simulink model "regulator_dyskretny"  (R2013b)
settings: Solver=ode3  StartTime=0.0  StopTime=500  FixedStep=0.1  RelTol=1e-3
values from neighbouring files (symbols this model uses):
  a = 31    [charakterystyka_pompa.m]    (also in charakterystyka_pompa_sterownik.m; dane14listopad.mat; danePompa.mat; pomiary.m)
  b = 40    [charakterystyki_zawory_reczne.m]    (also in daneZawory_cz2.mat; pomiary.m; rhs.m)
  c = p(1)    [cel.m]    (also in charakterystyki_zawory_reczne.m = 10; daneZawory_cz2.mat = 10; identyfikacja_parametrow.m = 10; identyfikacja_zawor2.m = 10)
  C1 = q/sqrt(H1pp)    [linearyzacja_analitycznie.m]    (also in wskaznikZawor1.m = parametry(1))
  C2 = q/sqrt(H2pp)    [linearyzacja_analitycznie.m]    (also in wskaznikZawor2.m = parametry(1))
  C3 = q/sqrt(H3pp)    [linearyzacja_analitycznie.m]    (also in wskaznikZawor3.m = parametry(1))
  H2max = 40    [charakterystyki_zawory_reczne.m]    (also in daneZawory_cz2.mat; pomiary.m)
  K = [0.0311 0.0151 0.0068]    [testy_regulatora.m]    (also in wagiLQ.m = K_par)
  R = 40    [charakterystyki_zawory_reczne.m]    (also in daneZawory_cz2.mat; nastawyLQ.m; pomiary.m; rhs.m)
  w = 5    [charakterystyka_pompa.m]    (also in charakterystyka_pompa_sterownik.m; dane14listopad.mat; danePompa.mat; pomiary.m)
  x = max(x,0)    [rhs.m]
settings Model: Creator=Michal  LastModifiedBy=Michal

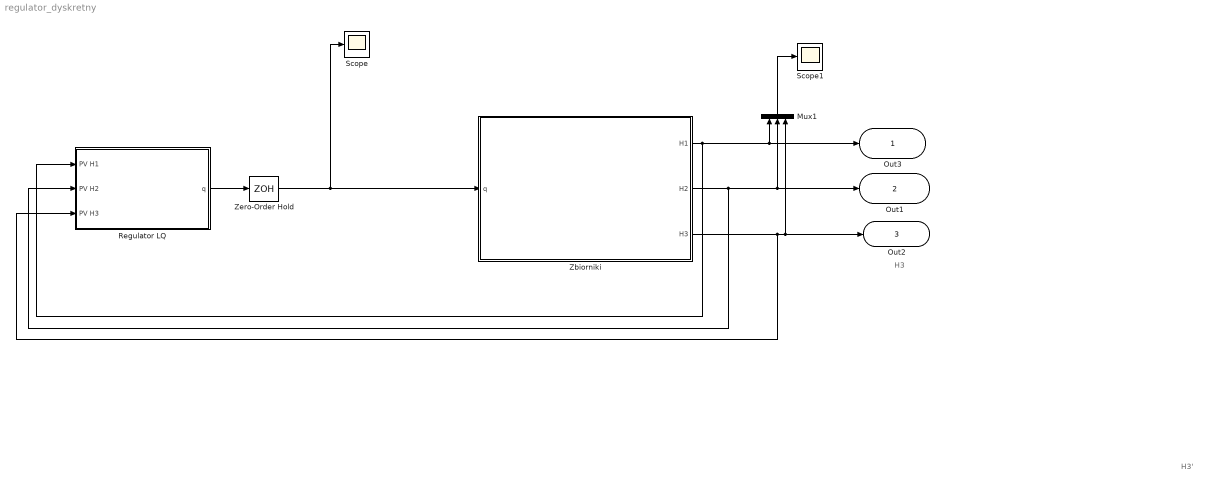
== system regulator_dyskretny ==
  note: H3
  note: H3'
  Mux1 : Mux  Inputs=3
  Regulator LQ : Subsystem
  Scope : Scope
      settings: TimeRange=500  SaveName=q_lqr
  Scope1 : Scope
      settings: TimeRange=500  YMin=-300000  YMax=50000  SaveName=H_lqr
  Zbiorniki : Subsystem
  Zero-Order Hold : ZeroOrderHold  SampleTime=0.1
  Out3 : Outport
  Out1 : Outport  Port=2
  Out2 : Outport  Port=3
  wires:
  Zbiorniki/3(H3) -> Regulator LQ/3(PV H3), Out2/1, Mux1/3
  Zbiorniki/1(H1) -> Regulator LQ/1(PV H1), Mux1/1, Out3/1
  Zbiorniki/2(H2) -> Regulator LQ/2(PV H2), Mux1/2, Out1/1
  Mux1/1 -> Scope1/1
  Regulator LQ/1(q) -> Zero-Order Hold/1
  Zero-Order Hold/1 -> Scope/1, Zbiorniki/1(q)

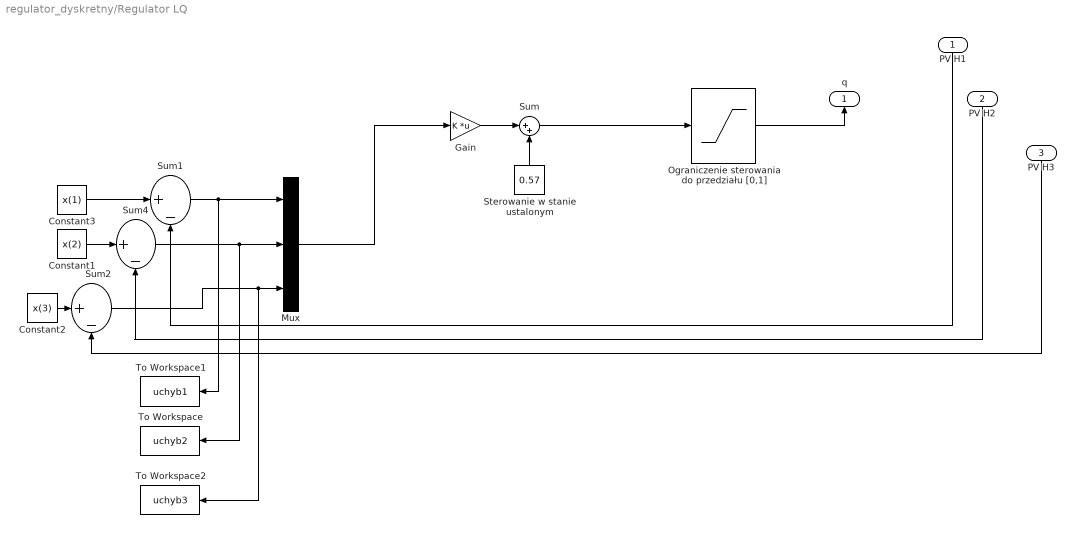
== system regulator_dyskretny/Regulator LQ ==
  PV H1 : Inport
  PV H2 : Inport  Port=2
  PV H3 : Inport  Port=3
  Constant1 : Constant  Value=x(2)
  Constant2 : Constant  Value=x(3)
  Constant3 : Constant  Value=x(1)
  Gain : Gain  Gain=K  Multiplication=Matrix(K*u)
  Mux : Mux  Inputs=3
  Ograniczenie sterowania do przedziału [0,1] : Saturate  UpperLimit=1  LowerLimit=0
  Sterowanie w stanie ustalonym : Constant  Value=0.57
  Sum : Sum  Inputs=|++
  Sum1 : Sum  Inputs=|+-
  Sum2 : Sum  Inputs=|+-
  Sum4 : Sum  Inputs=|+-
  To Workspace : ToWorkspace  VariableName=uchyb2  SampleTime=-1  SaveFormat=Structure With Time
  To Workspace1 : ToWorkspace  VariableName=uchyb1  SampleTime=-1  SaveFormat=Structure With Time
  To Workspace2 : ToWorkspace  VariableName=uchyb3  SampleTime=-1  SaveFormat=Structure With Time
  q : Outport
  wires:
  PV H1/1 -> Sum1/2
  PV H3/1 -> Sum2/2
  PV H2/1 -> Sum4/2
  Sum1/1 -> To Workspace1/1, Mux/1
  Sum2/1 -> To Workspace2/1, Mux/3
  Sum4/1 -> To Workspace/1, Mux/2
  Constant2/1 -> Sum2/1
  Constant1/1 -> Sum4/1
  Constant3/1 -> Sum1/1
  Sterowanie w stanie ustalonym/1 -> Sum/2
  Ograniczenie sterowania do przedziału [0,1]/1 -> q/1
  Sum/1 -> Ograniczenie sterowania do przedziału [0,1]/1
  Gain/1 -> Sum/1
  Mux/1 -> Gain/1

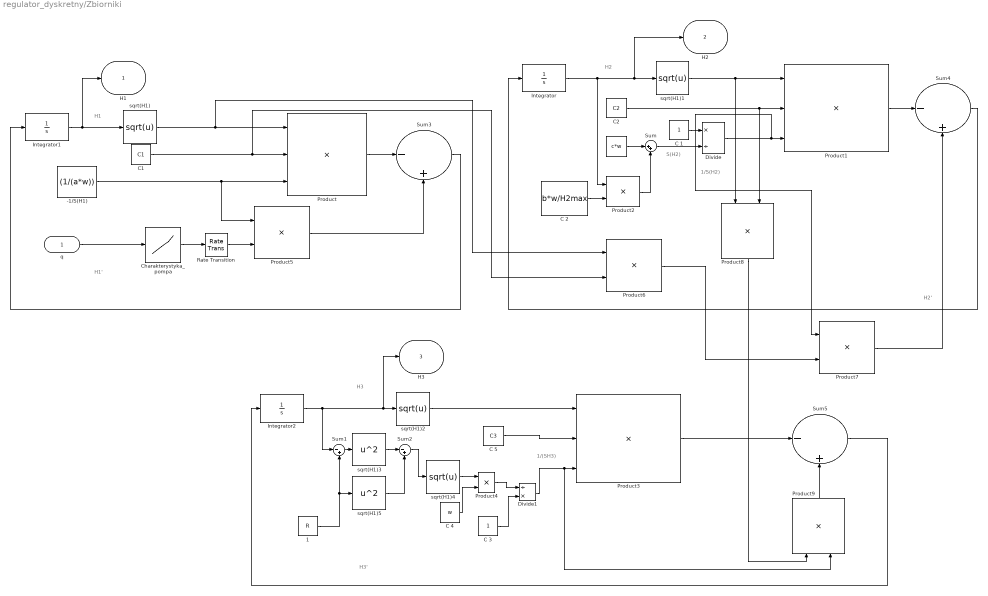
== system regulator_dyskretny/Zbiorniki ==
  note: H1
  note: 1/S(H2)
  note: S(H2)
  note: H2'
  note: H2
  note: 1/(SH3)
  note: H3
  note: H1'
  note: H3'
  q : Inport
  " " : Constant  Value=c*w
  " 1" : Constant  Value=R
  -1/S(H1) : Constant  Value=(1/(a*w))
  C 1 : Constant
  C 2 : Constant  Value=b*w/H2max
  C 3 : Constant
  C 4 : Constant  Value=w
  C 5 : Constant  Value=C3
  "C1 " : Constant  Value=C1
  "C2 " : Constant  Value=C2
  Charakterystyka_pompa : Lookup_n-D  NumberOfTableDimensions=1  BreakpointsForDimension1="[0.180000000000000\t0.181000000000000\t0.182000000000000\t0.183000000000000\t0.184000000000000\t0.185000000000000\t0.186000000000000\t0.187000000000000\t0.188000000000000\t0.189000000000000\t0.190000000000000\t0.191000000000000\t0.192000000000000\t0.193000000000000\t0.194000000000000\t0.195000000000000\t0.196000000000000\t0.197000000000000\t0.198000000000000\t0.199000000000000\t0.200000000000000\t0.201000000000000\t0.202000000000000\t0.203000000000000\t0.204000000000000\t0.205000000000000\t0.206000000000000\t0.207000000000000\t0.208000000000000\t0.209000000000000\t0.210000000000000\t0.211000000000000\t0.212000000000000\t0.213000000000000\t0.214000000000000\t0.215000000000000\t0.216000000000000\t0.217000000000000\t0.218000000000000\t0.219000000000000\t0.220000000000000\t0.221000000000000\t0.222000000000000\t0.223000000000000\t0.224000000000000\t0.225000000000000\t0.226000000000000\t0.227000000000000\t0.228000000000000\t0.229000000000000\t0.230000000000000\t0.231000000000000\t0.232000000000000\t0.233000000000000\t0.234000000000000\t0.235000000000000\t0.236000000000000\t0.237000000000000\t0.238000000000000\t0.239000000000000\t0.240000000000000\t0.241000000000000\t0.242000000000000\t0.243000000000000\t0.244000000000000\t0.245000000000000\t0.246000000000000\t0.247000000000000\t0.248000000000000\t0.249000000000000\t0.250000000000000\t0.251000000000000\t0.252000000000000\t0.253000000000000\t0.254000000000000\t0.255000000000000\t0.256000000000000\t0.257000000000000\t0.258000000000000\t0.259000000000000\t0.260000000000000\t0.261000000000000\t0.262000000000000\t0.263000000000000\t0.264000000000000\t0.265000000000000\t0.266000000000000\t0.267000000000000\t0.268000000000000\t0.269000000000000\t0.270000000000000\t0.271000000000000\t0.272000000000000\t0.273000000000000\t0.274000000000000\t0.275000000000000\t0.276000000000000\t0.277000000000000\t0.278000000000000\t0.279000000000000\t0.280000000000000\t0.281000000000000\t0.282000000000000\t0.283000000000000\t0.284000000000000\t0.285000000000000\t0.286000000000000\t0.287000000000000\t0.288000000000000\t0.289000000000000\t0.290000000000000\t0.291000000000000\t0.292000000000000\t0.293000000000000\t0.294000000000000\t0.295000000000000\t0.296000000000000\t0.297000000000000\t0.298000000000000\t0.299000000000000\t0.300000000000000\t0.301000000000000\t0.302000000000000\t0.303000000000000\t0.304000000000000\t0.305000000000000\t0.306000000000000\t0.307000000000000\t0.308000000000000\t0.309000000000000\t0.310000000000000\t0.311000000000000\t0.312000000000000\t0.313000000000000\t0.314000000000000\t0.315000000000000\t0.316000000000000\t0.317000000000000\t0.318000000000000\t0.319000000000000\t0.320000000000000\t0.321000000000000\t0.322000000000000\t0.323000000000000\t0.324000000000000\t0.325000000000000\t0.326000000000000\t0.327000000000000\t0.328000000000000\t0.329000000000000\t0.330000000000000\t0.331000000000000\t0.332000000000000\t0.333000000000000\t0.334000000000000\t0.335000000000000\t0.336000000000000\t0.337000000000000\t0.338000000000000\t0.339000000000000\t0.340000000000000\t0.341000000000000\t0.342000000000000\t0.343000000000000\t0.344000000000000\t0.345000000000000\t0.346000000000000\t0.347000000000000\t0.348000000000000\t0.349000000000000\t0.350000000000000\t0.351000000000000\t0.352000000000000\t0.353000000000000\t0.354000000000000\t0.355000000000000\t0.356000000000000\t0.357000000000000\t0.358000000000000\t0.359000000000000\t0.360000000000000\t0.361000000000000\t0.362000000000000\t0.363000000000000\t0.364000000000000\t0.365000000000000\t0.366000000000000\t0.367000000000000\t0.368000000000000\t0.369000000000000\t0.370000000000000\t0.371000000000000\t0.372000000000000\t0.373000000000000\t0.374000000000000\t0.375000000000000\t0.376000000000000\t0.377000000000000\t0.378000000000000\t0.379000000000000\t0.380000000000000\t0.381000000000000\t0.382000000000000\t0.383000000000000\t0.384000000000000\t0.385000000000000\t0.386000000000000\t0.387000000000000\t0.388000000000000\t0.389000000000000\t0.390000000000000\t0.391000000000000\t0.392000000000000\t0.393000000000000\t0.394000000000000\t0.395000000000000\t0.396000000000000\t0.397000000000000\t0.398000000000000\t0.399000000000000\t0.400000000000000\t0.401000000000000\t0.402000000000000\t0.403000000000000\t0.404000000000000\t0.405000000000000\t0.406000000000000\t0.407000000000000\t0.408000000000000\t0.409000000000000\t0.410000000000000\t0.411000000000000\t0.412000000000000\t0.413000000000000\t0.414000000000000\t0.415000000000000\t0.416000000000000\t0.417000000000000\t0.418000000000000\t0.419000000000000\t0.420000000000000\t0.421000000000000\t0.422000000000000\t0.423000000000000\t0.424000000000000\t0.425000000000000\t0.426000000000000\t0.427000000000000\t0.428000000000000\t0.429000000000000\t0.430000000000000\t0.431000000000000\t0.432000000000000\t0.433000000000000\t0.434000000000000\t0.435000000000000\t0.436000000000000\t0.437000000000000\t0.438000000000000\t0.439000000000000\t0.440000000000000\t0.441000000000000\t0.442000000000000\t0.443000000000000\t0.444000000000000\t0.445000000000000\t0.446000000000000\t0.447000000000000\t0.448000000000000\t0.449000000000000\t0.450000000000000\t0.451000000000000\t0.452000000000000\t0.453000000000000\t0.454000000000000\t0.455000000000000\t0.456000000000000\t0.457000000000000\t0.458000000000000\t0.459000000000000\t0.460000000000000\t0.461000000000000\t0.462000000000000\t0.463000000000000\t0.464000000000000\t0.465000000000000\t0.466000000000000\t0.467000000000000\t0.468000000000000\t0.469000000000000\t0.470000000000000\t0.471000000000000\t0.472000000000000\t0.473000000000000\t0.474000000000000\t0.475000000000000\t0.476000000000000\t0.477000000000000\t0.478000000000000\t0.479000000000000\t0.480000000000000\t0.481000000000000\t0.482000000000000\t0.483000000000000\t0.484000000000000\t0.485000000000000\t0.486000000000000\t0.487000000000000\t0.488000000000000\t0.489000000000000\t0.490000000000000\t0.491000000000000\t0.492000000000000\t0.493000000000000\t0.494000000000000\t0.495000000000000\t0.496000000000000\t0.497000000000000\t0.498000000000000\t0.499000000000000\t0.500000000000000\t0.501000000000000\t0.502000000000000\t0.503000000000000\t0.504000000000000\t0.505000000000000\t0.506000000000000\t0.507000000000000\t0.508000000000000\t0.509000000000000\t0.510000000000000\t0.511000000000000\t0.512000000000000\t0.513000000000000\t0.514000000000000\t0.515000000000000\t0.516000000000000\t0.517000000000000\t0.518000000000000\t0.519000000000000\t0.520000000000000\t0.521000000000000\t0.522000000000000\t0.523000000000000\t0.524000000000000\t0.525000000000000\t0.526000000000000\t0.527000000000000\t0.528000000000000\t0.529000000000000\t0.530000000000000\t0.531000000000000\t0.532000000000000\t0.533000000000000\t0.534000000000000\t0.535000000000000\t0.536000000000000\t0.537000000000000\t0.538000000000000\t0.539000000000000\t0.540000000000000\t0.541000000000000\t0.542000000000000\t0.543000000000000\t0.544000000000000\t0.545000000000000\t0.546000000000000\t0.547000000000000\t0.548000000000000\t0.549000000000000\t0.550000000000000\t0.551000000000000\t0.552000000000000\t0.553000000000000\t0.554000000000000\t0.555000000000000\t0.556000000000000\t0.557000000000000\t0.558000000000000\t0.559000000000000\t0.560000000000000\t0.561000000000000\t0.562000000000000\t0.563000000000000\t0.564000000000000\t0.565000000000000\t0.566000000000000\t0.567000000000000\t0.568000000000000\t0.569000000000000\t0.570000000000000\t0.571000000000000\t0.572000000000000\t0.573000000000000\t0.574000000000000\t0.575000000000000\t0.576000000000000\t0.577000000000000\t0.578000000000000\t0.579000000000000\t0.580000000000000\t0.581000000000000\t0.582000000000000\t0.583000000000000\t0.584000000000000\t0.585000000000000\t0.586000000000000\t0.587000000000000\t0.588000000000000\t0.589000000000000\t0.590000000000000\t0.591000000000000\t0.592000000000000\t0.593000000000000\t0.594000000000000\t0.595000000000000\t0.596000000000000\t0.597000000000000\t0.598000000000000\t0.599000000000000\t0.600000000000000\t0.601000000000000\t0.602000000000000\t0.603000000000000\t0.604000000000000\t0.605000000000000\t0.606000000000000\t0.607000000000000\t0.608000000000000\t0.609000000000000\t0.610000000000000\t0.611000000000000\t0.612000000000000\t0.613000000000000\t0.614000000000000\t0.615000000000000\t0.616000000000000\t0.617000000000000\t0.618000000000000\t0.619000000000000\t0.620000000000000\t0.621000000000000\t0.622000000000000\t0.623000000000000\t0.624000000000000\t0.625000000000000\t0.626000000000000\t0.627000000000000\t0.628000000000000\t0.629000000000000\t0.630000000000000\t0.631000000000000\t0.632000000000000\t0.633000000000000\t0.634000000000000\t0.635000000000000\t0.636000000000000\t0.637000000000000\t0.638000000000000\t0.639000000000000\t0.640000000000000\t0.641000000000000\t0.642000000000000\t0.643000000000000\t0.644000000000000\t0.645000000000000\t0.646000000000000\t0.647000000000000\t0.648000000000000\t0.649000000000000\t0.650000000000000\t0.651000000000000\t0.652000000000000\t0.653000000000000\t0.654000000000000\t0.655000000000000\t0.656000000000000\t0.657000000000000\t0.658000000000000\t0.659000000000000\t0.660000000000000\t0.661000000000000\t0.662000000000000\t0.663000000000000\t0.664000000000000\t0.665000000000000\t0.666000000000000\t0.667000000000000\t0.668000000000000\t0.669000000000000\t0.670000000000000\t0.671000000000000\t0.672000000000000\t0.673000000000000\t0.674000000000000\t0.675000000000000\t0.676000000000000\t0.677000000000000\t0.678000000000000\t0.679000000000000\t0.680000000000000\t0.681000000000000\t0.682000000000000\t0.683000000000000\t0.684000000000000\t0.685000000000000\t0.686000000000000\t0.687000000000000\t0.688000000000000\t0.689000000000000\t0.690000000000000\t0.691000000000000\t0.692000000000000\t0.693000000000000\t0.694000000000000\t0.695000000000000\t0.696000000000000\t0.697000000000000\t0.698000000000000\t0.699000000000000\t0.700000000000000\t0.701000000000000\t0.702000000000000\t0.703000000000000\t0.704000000000000\t0.705000000000000\t0.706000000000000\t0.707000000000000\t0.708000000000000\t0.709000000000000\t0.710000000000000\t0.711000000000000\t0.712000000000000\t0.713000000000000\t0.714000000000000\t0.715000000000000\t0.716000000000000\t0.717000000000000\t0.718000000000000\t0.719000000000000\t0.720000000000000\t0.721000000000000\t0.722000000000000\t0.723000000000000\t0.724000000000000\t0.725000000000000\t0.726000000000000\t0.727000000000000\t0.728000000000000\t0.729000000000000\t0.730000000000000\t0.731000000000000\t0.732000000000000\t0.733000000000000\t0.734000000000000\t0.735000000000000\t0.736000000000000\t0.737000000000000\t0.738000000000000\t0.739000000000000\t0.740000000000000\t0.741000000000000\t0.742000000000000\t0.743000000000000\t0.744000000000000\t0.745000000000000\t0.746000000000000\t0.747000000000000\t0.748000000000000\t0.749000000000000\t0.750000000000000\t0.751000000000000\t0.752000000000000\t0.753000000000000\t0.754000000000000\t0.755000000000000\t0.756000000000000\t0.757000000000000\t0.758000000000000\t0.759000000000000\t0.760000000000000\t0.761000000000000\t0.762000000000000\t0.763000000000000\t0.764000000000000\t0.765000000000000\t0.766000000000000\t0.767000000000000\t0.768000000000000\t0.769000000000000\t0.770000000000000\t0.771000000000000\t0.772000000000000\t0.773000000000000\t0.774000000000000\t0.775000000000000\t0.776000000000000\t0.777000000000000\t0.778000000000000\t0.779000000000000\t0.780000000000000\t0.781000000000000\t0.782000000000000\t0.783000000000000\t0.784000000000000\t0.785000000000000\t0.786000000000000\t0.787000000000000\t0.788000000000000\t0.789000000000000\t0.790000000000000\t0.791000000000000\t0.792000000000000\t0.793000000000000\t0.794000000000000\t0.795000000000000\t0.796000000000000\t0.797000000000000\t0.798000000000000\t0.799000000000000\t0.800000000000000\t0.801000000000000\t0.802000000000000\t0.803000000000000\t0.804000000000000\t0.805000000000000\t0.806000000000000\t0.807000000000000\t0.808000000000000\t0.809000000000000\t0.810000000000000\t0.811000000000000\t0.812000000000000\t0.813000000000000\t0.814000000000000\t0.815000000000000\t0.816000000000000\t0.817000000000000\t0.818000000000000\t0.819000000000000\t0.820000000000000\t0.821000000000000\t0.822000000000000\t0.823000000000000\t0.824000000000000\t0.825000000000000\t0.826000000000000\t0.827000000000000\t0.828000000000000\t0.829000000000000\t0.830000000000000\t0.831000000000000\t0.832000000000000\t0.833000000000000\t0.834000000000000\t0.835000000000000\t0.836000000000000\t0.837000000000000\t0.838000000000000\t0.839000000000000\t0.840000000000000\t0.841000000000000\t0.842000000000000\t0.843000000000000\t0.844000000000000\t0.845000000000000\t0.846000000000000\t0.847000000000000\t0.848000000000000\t0.849000000000000\t0.850000000000000\t0.851000000000000\t0.852000000000000\t0.853000000000000\t0.854000000000000\t0.855000000000000\t0.856000000000000\t0.857000000000000\t0.858000000000000\t0.859000000000000\t0.860000000000000\t0.861000000000000\t0.862000000000000\t0.863000000000000\t0.864000000000000\t0.865000000000000\t0.866000000000000\t0.867000000000000\t0.868000000000000\t0.869000000000000\t0.870000000000000\t0.871000000000000\t0.872000000000000\t0.873000000000000\t0.874000000000000\t0.875000000000000\t0.876000000000000\t0.877000000000000\t0.878000000000000\t0.879000000000000\t0.880000000000000\t0.881000000000000\t0.882000000000000\t0.883000000000000\t0.884000000000000\t0.885000000000000\t0.886000000000000\t0.887000000000000\t0.888000000000000\t0.889000000000000\t0.890000000000000\t0.891000000000000\t0.892000000000000\t0.893000000000000\t0.894000000000000\t0.895000000000000\t0.896000000000000\t0.897000000000000\t0.898000000000000\t0.899000000000000\t0.900000000000000\t0.901000000000000\t0.902000000000000\t0.903000000000000\t0.904000000000000\t0.905000000000000\t0.906000000000000\t0.907000000000000\t0.908000000000000\t0.909000000000000\t0.910000000000000\t0.911000000000000\t0.912000000000000\t0.913000000000000\t0.914000000000000\t0.915000000000000\t0.916000000000000\t0.917000000000000\t0.918000000000000\t0.919000000000000\t0.920000000000000\t0.921000000000000\t0.922000000000000\t0.923000000000000\t0.924000000000000\t0.925000000000000\t0.926000000000000\t0.927000000000000\t0.928000000000000\t0.929000000000000\t0.930000000000000\t0.931000000000000\t0.932000000000000\t0.933000000000000\t0.934000000000000\t0.935000000000000\t0.936000000000000\t0.937000000000000\t0.938000000000000\t0.939000000000000\t0.940000000000000\t0.941000000000000\t0.942000000000000\t0.943000000000000\t0.944000000000000\t0.945000000000000\t0.946000000000000\t0.947000000000000\t0.948000000000000\t0.949000000000000\t0.950000000000000\t0.951000000000000\t0.952000000000000\t0.953000000000000\t0.954000000000000\t0.955000000000000\t0.956000000000000\t0.957000000000000\t0.958000000000000\t0.959000000000000\t0.960000000000000\t0.961000000000000\t0.962000000000000\t0.963000000000000\t0.964000000000000\t0.965000000000000\t0.966000000000000\t0.967000000000000\t0.968000000000000\t0.969000000000000\t0.970000000000000\t0.971000000000000\t0.972000000000000\t0.973000000000000\t0.974000000000000\t0.975000000000000\t0.976000000000000\t0.977000000000000\t0.978000000000000\t0.979000000000000\t0.980000000000000\t0.981000000000000\t0.982000000000000\t0.983000000000000\t0.984000000000000\t0.985000000000000\t0.986000000000000\t0.987000000000000\t0.988000000000000\t0.989000000000000\t0.990000000000000\t0.991000000000000\t0.992000000000000\t0.993000000000000\t0.994000000000000\t0.995000000000000\t0.996000000000000\t0.997000000000000\t0.998000000000000\t0.999000000000000\t1]"  Table="[12.0028336476540\t12.3293606666216\t12.6550486652732\t12.9798992380227\t13.3039139792839\t13.6270944834709\t13.9494423449973\t14.2709591582772\t14.5916465177244\t14.9115060177528\t15.2305392527763\t15.5487478172088\t15.8661333054640\t16.1826973119561\t16.4984414310987\t16.8133672573059\t17.1274763849915\t17.4407704085693\t17.7532509224533\t18.0649195210574\t18.3757777987953\t18.6858273500811\t18.9950697693286\t19.3035066509517\t19.6111395893642\t19.9179701789801\t20.2240000142132\t20.5292306894775\t20.8336637991868\t21.1373009377549\t21.4401436995959\t21.7421936791235\t22.0434524707516\t22.3439216688942\t22.6436028679651\t22.9424976623782\t23.2406076465474\t23.5379344148866\t23.8344795618096\t24.1302446817304\t24.4252313690628\t24.7194412182207\t25.0128758236180\t25.3055367796686\t25.5974256807863\t25.8885441213852\t26.1788936958789\t26.4684759986814\t26.7572926242067\t27.0453451668686\t27.3326352210809\t27.6191643812576\t27.9049342418125\t28.1899463971596\t28.4742024417127\t28.7577039698856\t29.0404525760924\t29.3224498547468\t29.6036974002628\t29.8841968070542\t30.1639496695350\t30.4429575821190\t30.7212221392200\t30.9987449352520\t31.2755275646289\t31.5515716217645\t31.8268787010728\t32.1014503969676\t32.3752883038628\t32.6483940161723\t32.9207691283099\t33.1924152346896\t33.4633339297253\t33.7335268078307\t34.0029954634199\t34.2717414909067\t34.5397664847049\t34.8070720392286\t35.0736597488914\t35.3395312081074\t35.6046880112905\t35.8691317528544\t36.1328640272131\t36.3958864287805\t36.6582005519705\t36.9198079911969\t37.1807103408736\t37.4409091954146\t37.7004061492336\t37.9592027967446\t38.2173007323615\t38.4747015504981\t38.7314068455684\t38.9874182119862\t39.2427372441654\t39.4973655365200\t39.7513046834636\t40.0045562794104\t40.2571219187741\t40.5090031959686\t40.7602017054078\t41.0107190415057\t41.2605567986760\t41.5097165713327\t41.7581999538896\t42.0060085407607\t42.2531439263599\t42.4996077051009\t42.7454014713977\t42.9905268196642\t43.2349853443143\t43.4787786397618\t43.7219083004207\t43.9643759207047\t44.2061830950279\t44.4473314178040\t44.6878224834471\t44.9276578863709\t45.1668392209893\t45.4053680817163\t45.6432460629656\t45.8804747591513\t46.1170557646872\t46.3529906739871\t46.5882810814650\t46.8229285815347\t47.0569347686101\t47.2903012371052\t47.5230295814337\t47.7551213960096\t47.9865782752468\t48.2174018135591\t48.4475936053605\t48.6771552450647\t48.9060883270858\t49.1343944458375\t49.3620751957338\t49.5891321711886\t49.8155669666157\t50.0413811764291\t50.2665763950425\t50.4911542168699\t50.7151162363253\t50.9384640478223\t51.1611992457751\t51.3833234245973\t51.6048381787030\t51.8257451025060\t52.0460457904202\t52.2657418368594\t52.4848348362376\t52.7033263829687\t52.9212180714665\t53.1385114961448\t53.3552082514177\t53.5713099316990\t53.7868181314025\t54.0017344449422\t54.2160604667319\t54.4297977911855\t54.6429480127170\t54.8555127257401\t55.0674935246688\t55.2788920039170\t55.4897097578985\t55.6999483810273\t55.9096094677171\t56.1186946123820\t56.3272054094357\t56.5351434532922\t56.7425103383654\t56.9493076590691\t57.1555370098172\t57.3611999850236\t57.5662981791023\t57.7708331864670\t57.9748066015317\t58.1782200187102\t58.3810750324164\t58.5833732370643\t58.7851162270677\t58.9863055968404\t59.1869429407965\t59.3870298533496\t59.5865679289139\t59.7855587619030\t59.9840039467310\t60.1819050778117\t60.3792637495589\t60.5760815563866\t60.7723600927087\t60.9681009529389\t61.1633057314914\t61.3579760227798\t61.5521134212181\t61.7457195212202\t61.9387959171999\t62.1313442035712\t62.3233659747479\t62.5148628251439\t62.7058363491732\t62.8962881412495\t63.0862197957868\t63.2756329071989\t63.4645290698998\t63.6529098783032\t63.8407769268232\t64.0281318098736\t64.2149761218683\t64.4013114572211\t64.5871394103460\t64.7724615756568\t64.9572795475674\t65.1415949204918\t65.3254092888437\t65.5087242470371\t65.6915413894858\t65.8738623106038\t66.0556886048049\t66.2370218665030\t66.4178636901120\t66.5982156700458\t66.7780794007183\t66.9574564765433\t67.1363484919347\t67.3147570413065\t67.4926837190724\t67.6701301196465\t67.8470978374425\t68.0235884668744\t68.1996036023560\t68.3751448383013\t68.5502137691241\t68.7248119892382\t68.8989410930576\t69.0726026749963\t69.2457983294680\t69.4185296508865\t69.5907982336660\t69.7626056722201\t69.9339535609629\t70.1048434943080\t70.2752770666696\t70.4452558724614\t70.6147815060973\t70.7838555619913\t70.9524796345572\t71.1206553182088\t71.2883842073601\t71.4556678964250\t71.6225079798173\t71.7889060519509\t71.9548637072397\t72.1203825400977\t72.2854641449386\t72.4501101161764\t72.6143220482249\t72.7781015354980\t72.9414501724097\t73.1043695533738\t73.2668612728042\t73.4289269251147\t73.5905681047193\t73.7517864060318\t73.9125834234662\t74.0729607514363\t74.2329199843560\t74.3924627166392\t74.5515905426997\t74.7103050569515\t74.8686078538084\t75.0265005276843\t75.1839846729932\t75.3410618841488\t75.4977337555651\t75.6540018816559\t75.8098678568353\t75.9653332755169\t76.1203997321148\t76.2750688210427\t76.4293421367147\t76.5832212735445\t76.7367078259461\t76.8898033883332\t77.0425095551200\t77.1948279207201\t77.3467600795475\t77.4983076260161\t77.6494721545398\t77.8002552595325\t77.9506585354079\t78.1006835765800\t78.2503319774628\t78.3996053324701\t78.5485052360157\t78.6970332825136\t78.8451910663776\t78.9929801820217\t79.1404022238596\t79.2874587863054\t79.4341514637729\t79.5804818506758\t79.7264515414283\t79.8720621304441\t80.0173152121371\t80.1622123809213\t80.3067552312104\t80.4509453574184\t80.5947843539591\t80.7382738152465\t80.8814153356944\t81.0242105097167\t81.1666609317274\t81.3087681961402\t81.4505338973690\t81.5919596298279\t81.7330469879306\t81.8737975660909\t82.0142129587229\t82.1542947602405\t82.2940445650573\t82.4334639675875\t82.5725545622448\t82.7113179434431\t82.8497557055963\t82.9878694431183\t83.1256607504231\t83.2631312219243\t83.4002824520361\t83.5371160351722\t83.6736335657465\t83.8098366381729\t83.9457268468653\t84.0813057862376\t84.2165750507037\t84.3515362346774\t84.4861909325726\t84.6205407388033\t84.7545872477833\t84.8883320539264\t85.0217767516467\t85.1549229353579\t85.2877721994739\t85.4203261384087\t85.5525863465760\t85.6845544183899\t85.8162319482642\t85.9476205306127\t86.0787217598494\t86.2095372303881\t86.3400685366427\t86.4703172730272\t86.6002850339553\t86.7299734138410\t86.8593840070982\t86.9885184081407\t87.1173782113825\t87.2459650112374\t87.3742804021192\t87.5023259784420\t87.6301033346195\t87.7576140650657\t87.8848597641944\t88.0118420264195\t88.1385624461550\t88.2650226178146\t88.3912241358123\t88.5171685945621\t88.6428575884776\t88.7682927119728\t88.8934755594617\t89.0184077253581\t89.1430908040759\t89.2675263900290\t89.3917160776312\t89.5156614612964\t89.6393641354386\t89.7628256944716\t89.8860477328093\t90.0090318448656\t90.1317796250543\t90.2542926677894\t90.3765725674847\t90.4986209185542\t90.6204393154117\t90.7420293524710\t90.8633926241461\t90.9845307248509\t91.1054452489992\t91.2261377910050\t91.3466099452821\t91.4668633062444\t91.5868994683057\t91.7067200258800\t91.8263265733812\t91.9457207052231\t92.0649040158197\t92.1838780995847\t92.3026445509322\t92.4212049642759\t92.5395609340298\t92.6577140546077\t92.7756659204236\t92.8934181258913\t93.0109722654247\t93.1283299334376\t93.2454927243441\t93.3624622325579\t93.4792400524930\t93.5958277785631\t93.7122270051823\t93.8284393267644\t93.9444663377232\t94.0603096324728\t94.1759708054268\t94.2914514509994\t94.4067531636042\t94.5218775376552\t94.6368261675664\t94.7516006477515\t94.8662025726245\t94.9806335365991\t95.0948951340895\t95.2089889595093\t95.3229166072726\t95.4366796717931\t95.5502797474848\t95.6637184287616\t95.7769973100373\t95.8901179857258\t96.0030820502411\t96.1158910979969\t96.2285467234072\t96.3410505208858\t96.4534040848468\t96.5656090097038\t96.6776668898708\t96.7895793197618\t96.9013478937905\t97.0129742063709\t97.1244598519169\t97.2358064248424\t97.3470155195611\t97.4580887304870\t97.5690276520341\t97.6798338786161\t97.7905090046470\t97.9010546245406\t98.0114723327109\t98.1217637235717\t98.2319303915369\t98.3419739310204\t98.4518959364360\t98.5616980021977\t98.6713817227194\t98.7809486924149\t98.8904005056981\t98.9997387569829\t99.1089650406832\t99.2180809512128\t99.3270880829858\t99.4359880304158\t99.5447823879168\t99.6534727499028\t99.7620607107876\t99.8705478649851\t99.9789358069090\t100.087226130973\t100.195420431592\t100.303520303179\t100.411527340148\t100.519443136913\t100.627269287888\t100.735007387487\t100.842659030123\t100.950225810211\t101.057709322165\t101.165111160397\t101.272432919323\t101.379676193356\t101.486842576910\t101.593933664398\t101.700951050235\t101.807896328835\t101.914771094612\t102.021576941979\t102.128315465350\t102.234988259139\t102.341596917760\t102.448143035627\t102.554628207154\t102.661054026755\t102.767422088843\t102.873733987833\t102.979991318137\t103.086195674172\t103.192348650349\t103.298451841083\t103.404506840788\t103.510515243878\t103.616478644767\t103.722398637868\t103.828276817595\t103.934114778363\t104.039914114585\t104.145676420675\t104.251403291047\t104.357096320115\t104.462757102293\t104.568387231994\t104.673988303633\t104.779561911623\t104.885109650378\t104.990633114312\t105.096133897840\t105.201613595374\t105.307073801330\t105.412516110120\t105.517942116158\t105.623353413859\t105.728751597636\t105.834138261904\t105.939515001075\t106.044883409565\t106.150245081787\t106.255601612154\t106.360954595081\t106.466305624981\t106.571656296269\t106.677008203358\t106.782362940663\t106.887722102596\t106.993087283572\t107.098460078006\t107.203842080310\t107.309234884898\t107.414640086185\t107.520059278585\t107.625494056511\t107.730946014377\t107.836416746596\t107.941907847584\t108.047420911754\t108.152957533519\t108.258519307294\t108.364107827493\t108.469724688528\t108.575371484815\t108.681049810768\t108.786761260799\t108.892507429323\t108.998289910753\t109.104110299505\t109.209970189991\t109.315871176625\t109.421814853822\t109.527802815995\t109.633836657558\t109.739917972925\t109.846048356509\t109.952229402726\t110.058462705988\t110.164749860710\t110.271092461305\t110.377492102187\t110.483950377770\t110.590468882469\t110.697049210696\t110.803692956867\t110.910401715394\t111.017177080691\t111.124020647173\t111.230934009253\t111.337918761346\t111.444976497865\t111.552108813223\t111.659317301836\t111.766603558117\t111.873969176479\t111.981415751336\t112.088944877103\t112.196558148193\t112.304257159021\t112.412043504000\t112.519918777543\t112.627884574066\t112.735942487981\t112.844094113703\t112.952341045645\t113.060684878222\t113.169127205847\t113.277669622934\t113.386313723897\t113.495061103150\t113.603913355107\t113.712872074182\t113.821938854788\t113.931115291340\t114.040402978251\t114.149803509936\t114.259318480807\t114.368949485279\t114.478698117767\t114.588565972683\t114.698554644442\t114.808665727457\t114.918900816143\t115.029261504913\t115.139749388181\t115.250366060362\t115.361113115868\t115.471992149115\t115.583004754515\t115.694152526482\t115.805437059431\t115.916859947776\t116.028422785930\t116.140127168307\t116.251974689321\t116.363966943386\t116.476105524916\t116.588392028324\t116.700828048025\t116.813415178433\t116.926155013961\t117.039049149023\t117.152099178034\t117.265306695406\t117.378673295554\t117.492200572892\t117.605890121834\t117.719743536793\t117.833762412184\t117.947948342420\t118.062302921915\t118.176827745084\t118.291524406339\t118.406394500095\t118.521439620766\t118.636661362766\t118.752061320508\t118.867641088407\t118.983402260876\t119.099346432329\t119.215475197180\t119.331790149843\t119.448292884731\t119.564984996260\t119.681868078842\t119.798943726892\t119.916213534823\t120.033679097049\t120.151342007984\t120.269203862043\t120.387266253638\t120.505530777184\t120.623999027095\t120.742672597784\t120.861553083666\t120.980642079154\t121.099941178663\t121.219451976605\t121.339176067396\t121.459115045448\t121.579270505176\t121.699644040994\t121.820237247315\t121.941051718554\t122.062089049124\t122.183350833439\t122.304838665913\t122.426554140960\t122.548498852994\t122.670674396429\t122.793082365678\t122.915724355156\t123.038601959276\t123.161716772453\t123.285070389099\t123.408664403630\t123.532500410458\t123.656580003998\t123.780904778664\t123.905476328870\t124.030296249029\t124.155366133555\t124.280687576863\t124.406262173366\t124.532091517477\t124.658177203612\t124.784520826183\t124.911123979605\t125.037988258292\t125.165115256657\t125.292506569114\t125.420163790077\t125.548088513961\t125.676282335178\t125.804746848143\t125.933483647270\t126.062494326973\t126.191780481665\t126.321343705761\t126.451185593673\t126.581307739817\t126.711711738606\t126.842399184454\t126.973371671775\t127.104630794982\t127.236178148490\t127.368015326712\t127.500143924063\t127.632565534956\t127.765281753805\t127.898294175024\t128.031604393027\t128.165214002228\t128.299124597040\t128.433337771878\t128.567855121155\t128.702678239286\t128.837808720683\t128.973248159762\t129.108998150936\t129.245060288619\t129.381436167224\t129.518127381166\t129.655135524859\t129.792462192716\t129.930108979151\t130.068077478578\t130.206369285412\t130.344985994065\t130.483929198952\t130.623200494487\t130.762801475083\t130.902733735155\t131.042998869116\t131.183598471381\t131.324534136362\t131.465807458475\t131.607420032132\t131.749373451749\t131.891669311737\t132.034309206513\t132.177294730489\t132.320627478079\t132.464309043697\t132.608341021758\t132.752725006674\t132.897462592860\t133.042555374730\t133.188004946698\t133.333812903177\t133.479980838582\t133.626510347325\t133.773403023822\t133.920660462486\t134.068284257731\t134.216276003971\t134.364637295619\t134.513369727090\t134.662474892798\t134.811954387156\t134.961809804578\t135.112042739478\t135.262654786270\t135.413647539368\t135.565022593186\t135.716781542138\t135.868925980637\t136.021457503097\t136.174377703933\t136.327688177558\t136.481390518386\t136.635486320831\t136.789977179307\t136.944864688228\t137.100150442007\t137.255836035059\t137.411923061797\t137.568413116636\t137.725307793989\t137.882608688269\t138.040317393892\t138.198435505270\t138.356964616819\t138.515906322950\t138.675262218080\t138.835033896620\t138.995222952986\t139.155830981591\t139.316859576849\t139.478310333174\t139.640184844980\t139.802484706680\t139.965211512689\t140.128366857420\t140.291952335288\t140.455969540706\t140.620420068088\t140.785305511848\t140.950627466400\t141.116387526157\t141.282587285534\t141.449228338945\t141.616312280803\t141.783840705522\t141.951815207517\t142.120237381201\t142.289108820987\t142.458431121290\t142.628205876525\t142.798434681103\t142.969119129440\t143.140260815950\t143.311861335046\t143.483922281142\t143.656445248652\t143.829431831989\t144.002883625569]"  InterpMethod=Cubic spline  ExtrapMethod=Cubic spline  InternalRulePriority=Speed  RndMeth=Simplest  InputSameDT=on
  Divide : Product  Inputs=*/
  Divide1 : Product  Inputs=/*
  Integrator : Integrator  InitialCondition=0.01
  Integrator1 : Integrator  InitialCondition=0.01
  Integrator2 : Integrator  InitialCondition=0.01
  Product : Product  Inputs=3
  Product1 : Product  Inputs=3
  Product{2,4..9} (7 alike) : Product
  Product3 : Product  Inputs=3
  Rate Transition : RateTransition  OutPortSampleTimeOpt=Multiple of input port sample time  OutPortSampleTimeMultiple=0.1
  Sum : Sum  Inputs=|++
  Sum{1..5} (5 alike) : Sum  Inputs=|-+
  sqrt(H1){,1..2,4} (4 alike) : Fcn  Expr=sqrt(u)
  sqrt(H1)3 : Fcn  Expr=u^2
  sqrt(H1)5 : Fcn  Expr=u^2
  H1 : Outport
  H2 : Outport  Port=2
  H3 : Outport  Port=3
  wires:
  Product1/1 -> Sum4/1
  Product/1 -> Sum3/1
  Product5/1 -> Sum3/2
  Sum4/1 -> Integrator/1
  Sum5/1 -> Integrator2/1
  Sum3/1 -> Integrator1/1
  Product7/1 -> Sum4/2
  Product6/1 -> Product7/2
  Integrator/1 -> Product2/1, H2/1, sqrt(H1)1/1
  Product9/1 -> Sum5/2
  sqrt(H1)/1 -> Product6/1, Product/1
  Integrator1/1 -> H1/1, sqrt(H1)/1
  -1/S(H1)/1 -> Product5/1, Product/3
  "C1 "/1 -> Product6/2, Product/2
  sqrt(H1)5/1 -> Sum2/2
  Divide1/1 -> Product9/2, Product3/3
  C 4/1 -> Product4/2
  Product4/1 -> Divide1/1
  C 3/1 -> Divide1/2
  C 5/1 -> Product3/2
  sqrt(H1)2/1 -> Product3/1
  " 1"/1 -> sqrt(H1)5/1, Sum1/2
  Sum2/1 -> sqrt(H1)4/1
  Sum1/1 -> sqrt(H1)3/1
  sqrt(H1)4/1 -> Product4/1
  sqrt(H1)3/1 -> Sum2/1
  Integrator2/1 -> H3/1, sqrt(H1)2/1, Sum1/1
  Product3/1 -> Sum5/1
  Divide/1 -> Product1/3, Product7/1
  C 1/1 -> Divide/1
  Sum/1 -> Divide/2
  Product2/1 -> Sum/2
  C 2/1 -> Product2/2
  " "/1 -> Sum/1
  "C2 "/1 -> Product1/2, Product8/2
  sqrt(H1)1/1 -> Product1/1, Product8/1
  Product8/1 -> Product9/1
  Charakterystyka_pompa/1 -> Rate Transition/1
  q/1 -> Charakterystyka_pompa/1
  Rate Transition/1 -> Product5/2
